simulink model "AttitudeDetermination"  (R2023a)
settings: Solver=VariableStepAuto  StartTime=0.0  StopTime=10.0  RelTol=1e-3
libraries: simulink_extras x3
settings Model: Creator=aan18022  LastModifiedBy=aan18022

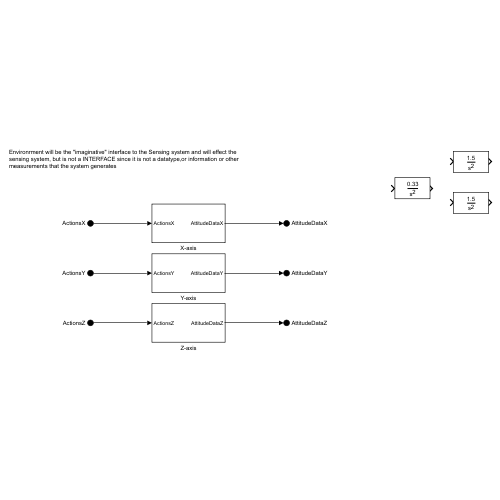
[thumbnail: Simulink's stored preview of the top-level diagram]
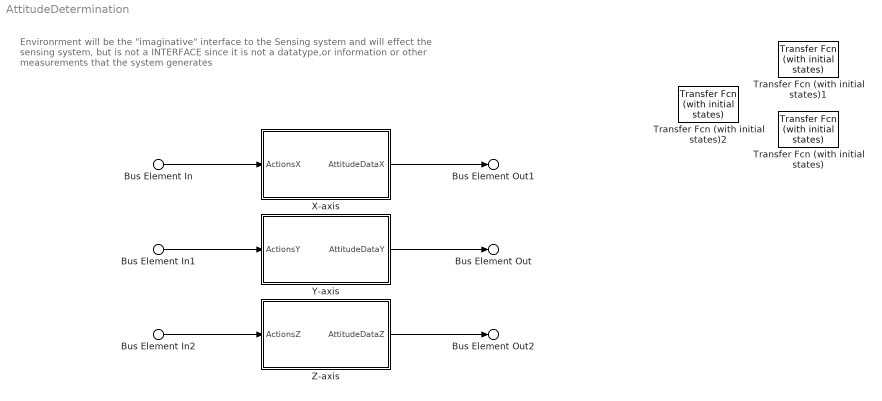
== system AttitudeDetermination ==
  note: Environrment will be the "imaginative" interface to the Sensing system and will effect the sensing system, but is not a INTERFACE since it is not a datatype,or information or other measurements that the system generates
  Bus Element In : Inport  PortName=ActionsX
  Bus Element In1 : Inport  Port=2  PortName=ActionsY
  Bus Element In2 : Inport  Port=3  PortName=ActionsZ
  Transfer Fcn (with initial states) : simulink_extras/Additional Linear/Transfer Fcn (with initial states)  N=[0.15*10]  D=[1,0,0]  X0=1
  Transfer Fcn (with initial states)1 : simulink_extras/Additional Linear/Transfer Fcn (with initial states)  N=[0.15*10]  D=[1,0,0]  X0=1
  Transfer Fcn (with initial states)2 : simulink_extras/Additional Linear/Transfer Fcn (with initial states)  N=[0.033*10]  D=[1,0,0]  X0=1
  X-axis : Subsystem
  Y-axis : Subsystem
  Z-axis : Subsystem
  Bus Element Out1 : Outport  PortName=AttitudeDataX
  Bus Element Out : Outport  Port=2  PortName=AttitudeDataY
  Bus Element Out2 : Outport  Port=3  PortName=AttitudeDataZ
  wires:
  Bus Element In/1 -> X-axis/1(ActionsX)
  Bus Element In1/1 -> Y-axis/1(ActionsY)
  Bus Element In2/1 -> Z-axis/1(ActionsZ)
  Z-axis/1(AttitudeDataZ) -> Bus Element Out2/1
  Y-axis/1(AttitudeDataY) -> Bus Element Out/1
  X-axis/1(AttitudeDataX) -> Bus Element Out1/1

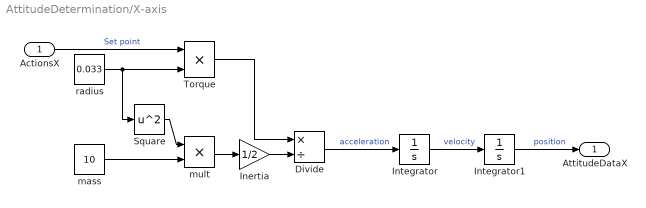
== system AttitudeDetermination/X-axis ==
  ActionsX : Inport
  Divide : Product  Inputs=*/
  Inertia : Gain  Gain=1/2
  Integrator : Integrator  InitialCondition=1
  Integrator1 : Integrator  InitialCondition=1
  Square : Math  Operator=square
  Torque : Product
  mass : Constant  Value=10
  mult : Product
  radius : Constant  Value=0.033
  AttitudeDataX : Outport
  wires:
  radius/1 -> Square/1, Torque/2
  Square/1 -> mult/1
  mult/1 -> Inertia/1
  Divide/1 -> Integrator/1  "acceleration"
  Integrator/1 -> Integrator1/1  "velocity"
  Torque/1 -> Divide/1
  mass/1 -> mult/2
  Inertia/1 -> Divide/2
  ActionsX/1 -> Torque/1  "Set point"
  Integrator1/1 -> AttitudeDataX/1  "position"

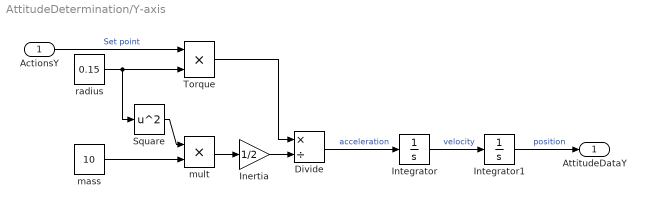
== system AttitudeDetermination/Y-axis ==
  ActionsY : Inport
  Divide : Product  Inputs=*/
  Inertia : Gain  Gain=1/2
  Integrator : Integrator  InitialCondition=1
  Integrator1 : Integrator  InitialCondition=1
  Square : Math  Operator=square
  Torque : Product
  mass : Constant  Value=10
  mult : Product
  radius : Constant  Value=0.15
  AttitudeDataY : Outport
  wires:
  radius/1 -> Square/1, Torque/2
  Square/1 -> mult/1
  mult/1 -> Inertia/1
  Divide/1 -> Integrator/1  "acceleration"
  Integrator/1 -> Integrator1/1  "velocity"
  Torque/1 -> Divide/1
  mass/1 -> mult/2
  Inertia/1 -> Divide/2
  ActionsY/1 -> Torque/1  "Set point"
  Integrator1/1 -> AttitudeDataY/1  "position"

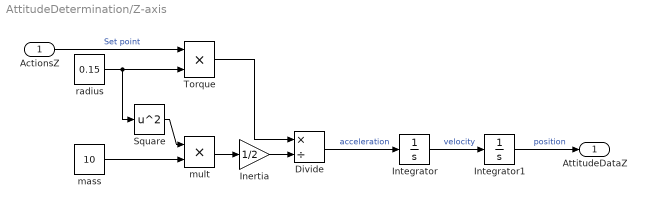
== system AttitudeDetermination/Z-axis ==
  ActionsZ : Inport
  Divide : Product  Inputs=*/
  Inertia : Gain  Gain=1/2
  Integrator : Integrator  InitialCondition=1
  Integrator1 : Integrator  InitialCondition=1
  Square : Math  Operator=square
  Torque : Product
  mass : Constant  Value=10
  mult : Product
  radius : Constant  Value=0.15
  AttitudeDataZ : Outport
  wires:
  radius/1 -> Square/1, Torque/2
  Square/1 -> mult/1
  mult/1 -> Inertia/1
  Divide/1 -> Integrator/1  "acceleration"
  Integrator/1 -> Integrator1/1  "velocity"
  Torque/1 -> Divide/1
  mass/1 -> mult/2
  Inertia/1 -> Divide/2
  ActionsZ/1 -> Torque/1  "Set point"
  Integrator1/1 -> AttitudeDataZ/1  "position"
